simulink library "pack_5p48s8p_4g4g4_Thr_library"  (R2026a)
settings: Solver=VariableStepAuto
undefined symbols (not defined in the file or in its folder): batt_5p48s_1g10g1_thr, batt_5p48s_4g4g4_thr, battery_builder_rtmsupport, gcbh, ModuleAssembly1, ModuleType1, plate_5p48s_4g4g4_thr, targets_5p48s8p_4g4g4_thr
libraries: $bdroot x24, batt_lib x17, cooling_system_components x10, pack_5p48s8p_4g4g4_Thr_lib x4, fl_lib x1
Description:
  | Copyright 2023-2026 The MathWorks, Inc.
settings Model: Creator=smiller  LastModifiedBy=smiller

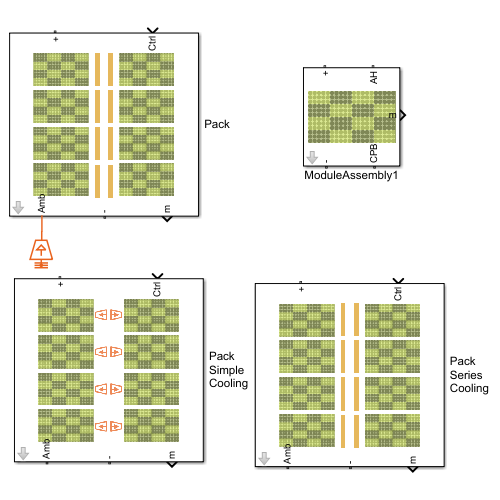
[thumbnail: Simulink's stored preview of the top-level diagram]
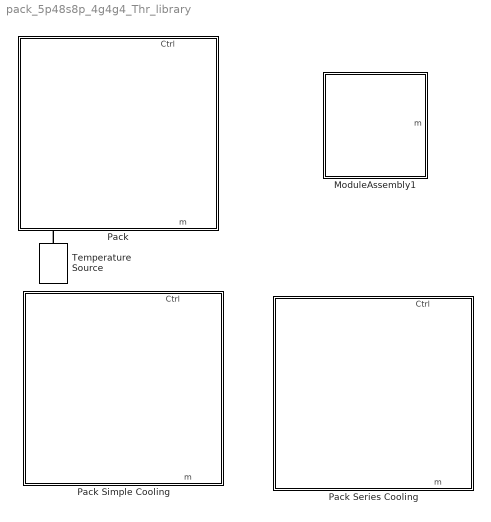
== system pack_5p48s8p_4g4g4_Thr_library ==
  ModuleAssembly1 : Subsystem  LoadFcn=battery_builder_rtmsupport('loadfcn',gcbh);  mask{Cell=ModuleType1, Targets=ModuleAssembly1, BatteryObj=batt_5p48s_1g10g1_thr}
      mask prompts: Cell "Cell Parameters"; Targets "Cell Targets"; BatteryObj "Battery Object"
      settings: PreCopyFcn=battery_builder_rtmsupport('precopyfcn',gcbh);  PreDeleteFcn=battery_builder_rtmsupport('predeletefcn',gcbh);  PortSchema="{\"entries\":[{\"content\":{\"sides\":[{\"content\":{\"connectorIds\":[\"LConn1\",\"LConn2\"]},\"type\":\"ConnectorPlacement.EquallySpacedRectSide\",\"uuid\":\"bc91a472-35c0-4041-89a6-b649b08794f0\"},{\"content\":{\"connectorIds\":[\"RConn1\",\"RConn2\"],\"side\":\"RIGHT\"},\"type\":\"ConnectorPlacement.EquallySpacedRectSide\",\"uuid\":\"4a390b53-12a2-4d2f-9537-abc76db307f8\"},{\"content\":{\"connectorIds\":[],\"side\":\"TOP\"},\"type\":\"ConnectorPlacement.EquallySpacedRectSide\",\"uuid\":\"1a7ed896-4ada-4d88-995c-c24bd39ee86b\"},{\"content\":{\"connectorIds\":[\"Out1\"],\"side\":\"BOTTOM\"},\"type\":\"ConnectorPlacement.EquallySpacedRectSide\",\"uuid\":\"e36c911b-adc9-44cf-bfab-32777b2ec35c\"}]},\"type\":\"ConnectorPlacement.EquallySpacedConnector\",\"uuid\":\"4e67d65b-f12d-4d00-91b0-7eadb0a42625\"}],\"packageUris\":[\"http://schema.mathworks.com/mf0/Connector/R2020b\"],\"version\":\"1.0\"}"
      mask Display: image('module_5p48s_4g4g4_IMAGE.png')
  Pack : Subsystem  LoadFcn=battery_builder_rtmsupport('loadfcn',gcbh);  mask{cell_param=ModuleType1, targets=targets_5p48s8p_4g4g4_thr, plate=plate_5p48s_4g4g4_thr, batt_obj=batt_5p48s_4g4g4_thr}
      mask prompts: cell_param "Cell Parameters"; targets "Cell Targets"; plate "Plate Parameters"; batt_obj "Battery Object"
      settings: PreCopyFcn=battery_builder_rtmsupport('precopyfcn',gcbh);  PreDeleteFcn=battery_builder_rtmsupport('predeletefcn',gcbh);
      mask Display: image('pack_5p48s8p_4g4g4_plate_IMAGE.png')
  Pack Series Cooling : Subsystem  LoadFcn=battery_builder_rtmsupport('loadfcn',gcbh);  mask{cell_param=ModuleType1, targets=targets_5p48s8p_4g4g4_thr, plate=plate_5p48s_4g4g4_thr, batt_obj=batt_5p48s_4g4g4_thr}
      mask prompts: cell_param "Cell Parameters"; targets "Cell Targets"; plate "Plate Parameters"; batt_obj "Battery Object"
      settings: PreCopyFcn=battery_builder_rtmsupport('precopyfcn',gcbh);  PreDeleteFcn=battery_builder_rtmsupport('predeletefcn',gcbh);
      mask Display: image('pack_5p48s8p_4g4g4_plate_IMAGE.png')
  Pack Simple Cooling : Subsystem  LoadFcn=battery_builder_rtmsupport('loadfcn',gcbh);  mask{cell_param=ModuleType1, targets=targets_5p48s8p_4g4g4_thr, plate=plate_5p48s_4g4g4_thr, batt_obj=batt_5p48s_4g4g4_thr, coolant_temp=[23 25]}
      mask prompts: cell_param "Cell Parameters"; targets "Cell Targets"; plate "Plate Parameters"; batt_obj "Battery Object"; coolant_temp "Coolant Temperature [In, Out] (degC)"
      settings: PreCopyFcn=battery_builder_rtmsupport('precopyfcn',gcbh);  PreDeleteFcn=battery_builder_rtmsupport('predeletefcn',gcbh);
      mask Display: image('pack_5p48s8p_4g4g4_bcnd_IMAGE.png')
  Temperature Source : fl_lib/Thermal/Thermal Sources/Temperature Source  temperature=298 K
  connections:
  Temperature Source/LConn1 -- Pack/RConn2

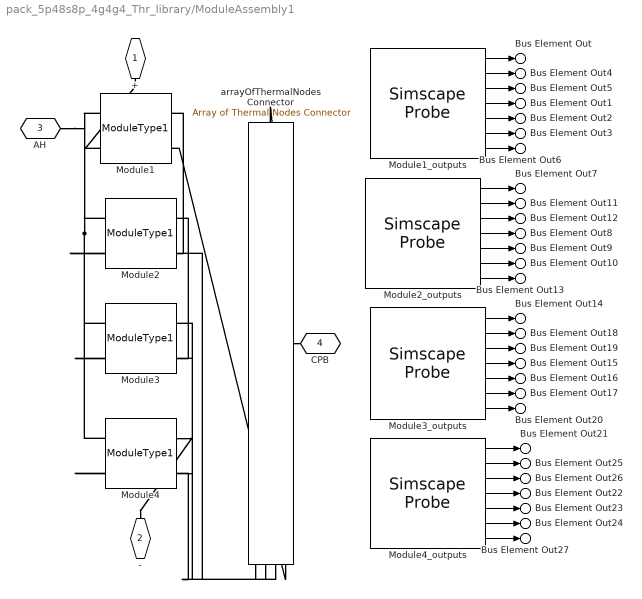
== system pack_5p48s8p_4g4g4_Thr_library/ModuleAssembly1 ==
  Module1 : pack_5p48s8p_4g4g4_Thr_lib/Modules/ModuleType1  BatteryCapacityCell=ModuleType1.BatteryCapacityCell A*hr  ExtrapolationMethodCell=simscape.enum.extrapolation.nearest  SOCBreakpointsCell=ModuleType1.SOCBreakpointsCell  TemperatureBreakpointsCell=ModuleType1.TemperatureBreakpointsCell K  OpenCircuitVoltageThermalCell=ModuleType1.OpenCircuitVoltageThermalCell V  VoltageRangeCell=ModuleType1.VoltageRangeCell V  ResistanceSOCBreakpointsCell=ModuleType1.ResistanceSOCBreakpointsCell  ResistanceTemperatureBreakpointsCell=ModuleType1.ResistanceTemperatureBreakpointsCell K  R0ThermalCell=ModuleType1.R0ThermalCell Ohm  BatteryThermalMassCell=ModuleType1.BatteryThermalMassCell J/K  CoolantResistance=Cell.CoolantResistance K/W  AmbientResistance=Cell.AmbientResistance K/W  socCell_specify=off  socCell_priority=High  socCell=repmat(1, 3, 1)  socCell_nominal_specify=off  socCell_nominal_value=1  socCell_nominal_unit=1  batteryVoltage_specify=off  batteryVoltage_priority=None  batteryVoltage=repmat(0, 3, 1) V  batteryVoltage_nominal_specify=off  batteryVoltage_nominal_value=1  batteryVoltage_nominal_unit=V  batteryCurrent_specify=off  batteryCurrent_priority=None  batteryCurrent=repmat(0, 3, 1) A  batteryCurrent_nominal_specify=off  batteryCurrent_nominal_value=1  batteryCurrent_nominal_unit=A  numCycles_specify=off  numCycles_priority=High  numCycles=repmat(0, 3, 1)  numCycles_nominal_specify=off  numCycles_nominal_value=1  numCycles_nominal_unit=1  batteryTemperature_specify=off  batteryTemperature_priority=High  batteryTemperature=repmat(298.15, 3, 1) K  batteryTemperature_nominal_specify=off  batteryTemperature_nominal_value=1  batteryTemperature_nominal_unit=K  vParallelAssembly_specify=on  vParallelAssembly_priority=None  vParallelAssembly=Targets.Module1.vParallelAssembly V  vParallelAssembly_nominal_specify=off  vParallelAssembly_nominal_value=1  vParallelAssembly_nominal_unit=V  socParallelAssembly_specify=on  socParallelAssembly_priority=None  socParallelAssembly=Targets.Module1.socParallelAssembly  socParallelAssembly_nominal_specify=off  socParallelAssembly_nominal_value=1  socParallelAssembly_nominal_unit=1
  Module1_outputs : SimscapeProbe  BoundBlock=1177  Variables="{\"batteryCurrent\":{\"Probing\":\"ON\"},\"batteryTemperature\":{\"Probing\":\"ON\"},\"batteryVoltage\":{\"Probing\":\"ON\"},\"iCell\":{\"Probing\":\"OFF\"},\"numCycles\":{\"Probing\":\"ON\"},\"numCyclesCell\":{\"Probing\":\"OFF\"},\"socCell\":{\"Probing\":\"ON\"},\"socParallelAssembly\":{\"Probing\":\"ON\"},\"temperatureCell\":{\"Probing\":\"OFF\"},\"vCell\":{\"Probing\":\"OFF\"},\"vParallelAssembly\":{\"Probing\":\"ON\"}}"
  Module2 : pack_5p48s8p_4g4g4_Thr_lib/Modules/ModuleType1  BatteryCapacityCell=ModuleType1.BatteryCapacityCell A*hr  ExtrapolationMethodCell=simscape.enum.extrapolation.nearest  SOCBreakpointsCell=ModuleType1.SOCBreakpointsCell  TemperatureBreakpointsCell=ModuleType1.TemperatureBreakpointsCell K  OpenCircuitVoltageThermalCell=ModuleType1.OpenCircuitVoltageThermalCell V  VoltageRangeCell=ModuleType1.VoltageRangeCell V  ResistanceSOCBreakpointsCell=ModuleType1.ResistanceSOCBreakpointsCell  ResistanceTemperatureBreakpointsCell=ModuleType1.ResistanceTemperatureBreakpointsCell K  R0ThermalCell=ModuleType1.R0ThermalCell Ohm  BatteryThermalMassCell=ModuleType1.BatteryThermalMassCell J/K  CoolantResistance=Cell.CoolantResistance K/W  AmbientResistance=Cell.AmbientResistance K/W  socCell_specify=off  socCell_priority=High  socCell=repmat(1, 3, 1)  socCell_nominal_specify=off  socCell_nominal_value=1  socCell_nominal_unit=1  batteryVoltage_specify=off  batteryVoltage_priority=None  batteryVoltage=repmat(0, 3, 1) V  batteryVoltage_nominal_specify=off  batteryVoltage_nominal_value=1  batteryVoltage_nominal_unit=V  batteryCurrent_specify=off  batteryCurrent_priority=None  batteryCurrent=repmat(0, 3, 1) A  batteryCurrent_nominal_specify=off  batteryCurrent_nominal_value=1  batteryCurrent_nominal_unit=A  numCycles_specify=off  numCycles_priority=High  numCycles=repmat(0, 3, 1)  numCycles_nominal_specify=off  numCycles_nominal_value=1  numCycles_nominal_unit=1  batteryTemperature_specify=off  batteryTemperature_priority=High  batteryTemperature=repmat(298.15, 3, 1) K  batteryTemperature_nominal_specify=off  batteryTemperature_nominal_value=1  batteryTemperature_nominal_unit=K  vParallelAssembly_specify=on  vParallelAssembly_priority=None  vParallelAssembly=Targets.Module2.vParallelAssembly V  vParallelAssembly_nominal_specify=off  vParallelAssembly_nominal_value=1  vParallelAssembly_nominal_unit=V  socParallelAssembly_specify=on  socParallelAssembly_priority=None  socParallelAssembly=Targets.Module2.socParallelAssembly  socParallelAssembly_nominal_specify=off  socParallelAssembly_nominal_value=1  socParallelAssembly_nominal_unit=1
  Module2_outputs : SimscapeProbe  BoundBlock=1178  Variables="{\"batteryCurrent\":{\"Probing\":\"ON\"},\"batteryTemperature\":{\"Probing\":\"ON\"},\"batteryVoltage\":{\"Probing\":\"ON\"},\"iCell\":{\"Probing\":\"OFF\"},\"numCycles\":{\"Probing\":\"ON\"},\"numCyclesCell\":{\"Probing\":\"OFF\"},\"socCell\":{\"Probing\":\"ON\"},\"socParallelAssembly\":{\"Probing\":\"ON\"},\"temperatureCell\":{\"Probing\":\"OFF\"},\"vCell\":{\"Probing\":\"OFF\"},\"vParallelAssembly\":{\"Probing\":\"ON\"}}"
  Module3 : pack_5p48s8p_4g4g4_Thr_lib/Modules/ModuleType1  BatteryCapacityCell=ModuleType1.BatteryCapacityCell A*hr  ExtrapolationMethodCell=simscape.enum.extrapolation.nearest  SOCBreakpointsCell=ModuleType1.SOCBreakpointsCell  TemperatureBreakpointsCell=ModuleType1.TemperatureBreakpointsCell K  OpenCircuitVoltageThermalCell=ModuleType1.OpenCircuitVoltageThermalCell V  VoltageRangeCell=ModuleType1.VoltageRangeCell V  ResistanceSOCBreakpointsCell=ModuleType1.ResistanceSOCBreakpointsCell  ResistanceTemperatureBreakpointsCell=ModuleType1.ResistanceTemperatureBreakpointsCell K  R0ThermalCell=ModuleType1.R0ThermalCell Ohm  BatteryThermalMassCell=ModuleType1.BatteryThermalMassCell J/K  CoolantResistance=Cell.CoolantResistance K/W  AmbientResistance=Cell.AmbientResistance K/W  socCell_specify=off  socCell_priority=High  socCell=repmat(1, 3, 1)  socCell_nominal_specify=off  socCell_nominal_value=1  socCell_nominal_unit=1  batteryVoltage_specify=off  batteryVoltage_priority=None  batteryVoltage=repmat(0, 3, 1) V  batteryVoltage_nominal_specify=off  batteryVoltage_nominal_value=1  batteryVoltage_nominal_unit=V  batteryCurrent_specify=off  batteryCurrent_priority=None  batteryCurrent=repmat(0, 3, 1) A  batteryCurrent_nominal_specify=off  batteryCurrent_nominal_value=1  batteryCurrent_nominal_unit=A  numCycles_specify=off  numCycles_priority=High  numCycles=repmat(0, 3, 1)  numCycles_nominal_specify=off  numCycles_nominal_value=1  numCycles_nominal_unit=1  batteryTemperature_specify=off  batteryTemperature_priority=High  batteryTemperature=repmat(298.15, 3, 1) K  batteryTemperature_nominal_specify=off  batteryTemperature_nominal_value=1  batteryTemperature_nominal_unit=K  vParallelAssembly_specify=on  vParallelAssembly_priority=None  vParallelAssembly=Targets.Module3.vParallelAssembly V  vParallelAssembly_nominal_specify=off  vParallelAssembly_nominal_value=1  vParallelAssembly_nominal_unit=V  socParallelAssembly_specify=on  socParallelAssembly_priority=None  socParallelAssembly=Targets.Module3.socParallelAssembly  socParallelAssembly_nominal_specify=off  socParallelAssembly_nominal_value=1  socParallelAssembly_nominal_unit=1
  Module3_outputs : SimscapeProbe  BoundBlock=1179  Variables="{\"batteryCurrent\":{\"Probing\":\"ON\"},\"batteryTemperature\":{\"Probing\":\"ON\"},\"batteryVoltage\":{\"Probing\":\"ON\"},\"iCell\":{\"Probing\":\"OFF\"},\"numCycles\":{\"Probing\":\"ON\"},\"numCyclesCell\":{\"Probing\":\"OFF\"},\"socCell\":{\"Probing\":\"ON\"},\"socParallelAssembly\":{\"Probing\":\"ON\"},\"temperatureCell\":{\"Probing\":\"OFF\"},\"vCell\":{\"Probing\":\"OFF\"},\"vParallelAssembly\":{\"Probing\":\"ON\"}}"
  Module4 : pack_5p48s8p_4g4g4_Thr_lib/Modules/ModuleType1  BatteryCapacityCell=ModuleType1.BatteryCapacityCell A*hr  ExtrapolationMethodCell=simscape.enum.extrapolation.nearest  SOCBreakpointsCell=ModuleType1.SOCBreakpointsCell  TemperatureBreakpointsCell=ModuleType1.TemperatureBreakpointsCell K  OpenCircuitVoltageThermalCell=ModuleType1.OpenCircuitVoltageThermalCell V  VoltageRangeCell=ModuleType1.VoltageRangeCell V  ResistanceSOCBreakpointsCell=ModuleType1.ResistanceSOCBreakpointsCell  ResistanceTemperatureBreakpointsCell=ModuleType1.ResistanceTemperatureBreakpointsCell K  R0ThermalCell=ModuleType1.R0ThermalCell Ohm  BatteryThermalMassCell=ModuleType1.BatteryThermalMassCell J/K  CoolantResistance=Cell.CoolantResistance K/W  AmbientResistance=Cell.AmbientResistance K/W  socCell_specify=off  socCell_priority=High  socCell=repmat(1, 3, 1)  socCell_nominal_specify=off  socCell_nominal_value=1  socCell_nominal_unit=1  batteryVoltage_specify=off  batteryVoltage_priority=None  batteryVoltage=repmat(0, 3, 1) V  batteryVoltage_nominal_specify=off  batteryVoltage_nominal_value=1  batteryVoltage_nominal_unit=V  batteryCurrent_specify=off  batteryCurrent_priority=None  batteryCurrent=repmat(0, 3, 1) A  batteryCurrent_nominal_specify=off  batteryCurrent_nominal_value=1  batteryCurrent_nominal_unit=A  numCycles_specify=off  numCycles_priority=High  numCycles=repmat(0, 3, 1)  numCycles_nominal_specify=off  numCycles_nominal_value=1  numCycles_nominal_unit=1  batteryTemperature_specify=off  batteryTemperature_priority=High  batteryTemperature=repmat(298.15, 3, 1) K  batteryTemperature_nominal_specify=off  batteryTemperature_nominal_value=1  batteryTemperature_nominal_unit=K  vParallelAssembly_specify=on  vParallelAssembly_priority=None  vParallelAssembly=Targets.Module4.vParallelAssembly V  vParallelAssembly_nominal_specify=off  vParallelAssembly_nominal_value=1  vParallelAssembly_nominal_unit=V  socParallelAssembly_specify=on  socParallelAssembly_priority=None  socParallelAssembly=Targets.Module4.socParallelAssembly  socParallelAssembly_nominal_specify=off  socParallelAssembly_nominal_value=1  socParallelAssembly_nominal_unit=1
  Module4_outputs : SimscapeProbe  BoundBlock=1180  Variables="{\"batteryCurrent\":{\"Probing\":\"ON\"},\"batteryTemperature\":{\"Probing\":\"ON\"},\"batteryVoltage\":{\"Probing\":\"ON\"},\"iCell\":{\"Probing\":\"OFF\"},\"numCycles\":{\"Probing\":\"ON\"},\"numCyclesCell\":{\"Probing\":\"OFF\"},\"socCell\":{\"Probing\":\"ON\"},\"socParallelAssembly\":{\"Probing\":\"ON\"},\"temperatureCell\":{\"Probing\":\"OFF\"},\"vCell\":{\"Probing\":\"OFF\"},\"vParallelAssembly\":{\"Probing\":\"ON\"}}"
  arrayOfThermalNodesConnector : batt_lib/Thermal/Array of Thermal Nodes Connector  numInputConnections=simscape.battery.enum.thermal.numArrayOfNodesConnections.four  concatenateDimension=2  complementaryDimensionsSize=1  inNode1NumElements=BatteryObj.Module(1).NumModels  inNode2NumElements=BatteryObj.Module(2).NumModels  inNode3NumElements=BatteryObj.Module(3).NumModels  inNode4NumElements=BatteryObj.Module(4).NumModels  inNode5NumElements=1  inNode6NumElements=1  inNode7NumElements=1  inNode8NumElements=1  inNode9NumElements=1  inNode10NumElements=1  inNode11NumElements=1  inNode12NumElements=1  inNode13NumElements=1  inNode14NumElements=1  inNode15NumElements=1  inNode16NumElements=1  inNode17NumElements=1  inNode18NumElements=1  inNode19NumElements=1  inNode20NumElements=1  inNode21NumElements=1  inNode22NumElements=1  inNode23NumElements=1  inNode24NumElements=1  inNode25NumElements=1  inNode26NumElements=1  inNode27NumElements=1  inNode28NumElements=1  inNode29NumElements=1  inNode30NumElements=1  inNode31NumElements=1  inNode32NumElements=1  inNode33NumElements=1  inNode34NumElements=1  inNode35NumElements=1  inNode36NumElements=1  inNode37NumElements=1  inNode38NumElements=1  inNode39NumElements=1  inNode40NumElements=1  inNode41NumElements=1  inNode42NumElements=1  inNode43NumElements=1  inNode44NumElements=1  inNode45NumElements=1  inNode46NumElements=1  inNode47NumElements=1  inNode48NumElements=1  inNode49NumElements=1  inNode50NumElements=1
  + : PMIOPort  Side=Left
  - : PMIOPort  Port=2  Side=Right
  AH : PMIOPort  Port=3  Side=Left
  CPB : PMIOPort  Port=4  Side=Right
  Bus Element Out : Outport  PortName=m  Element=i.M1
  Bus Element Out7 : Outport  PortName=m  Element=i.M2
  Bus Element Out14 : Outport  PortName=m  Element=i.M3
  Bus Element Out21 : Outport  PortName=m  Element=i.M4
  Bus Element Out1 : Outport  PortName=m  Element=cyc.M1
  Bus Element Out8 : Outport  PortName=m  Element=cyc.M2
  Bus Element Out15 : Outport  PortName=m  Element=cyc.M3
  Bus Element Out22 : Outport  PortName=m  Element=cyc.M4
  Bus Element Out2 : Outport  PortName=m  Element=socC.M1
  Bus Element Out9 : Outport  PortName=m  Element=socC.M2
  Bus Element Out16 : Outport  PortName=m  Element=socC.M3
  Bus Element Out23 : Outport  PortName=m  Element=socC.M4
  Bus Element Out3 : Outport  PortName=m  Element=socP.M1
  Bus Element Out10 : Outport  PortName=m  Element=socP.M2
  Bus Element Out17 : Outport  PortName=m  Element=socP.M3
  Bus Element Out24 : Outport  PortName=m  Element=socP.M4
  Bus Element Out4 : Outport  PortName=m  Element=T.M1
  Bus Element Out11 : Outport  PortName=m  Element=T.M2
  Bus Element Out18 : Outport  PortName=m  Element=T.M3
  Bus Element Out25 : Outport  PortName=m  Element=T.M4
  Bus Element Out5 : Outport  PortName=m  Element=vC.M1
  Bus Element Out12 : Outport  PortName=m  Element=vC.M2
  Bus Element Out19 : Outport  PortName=m  Element=vC.M3
  Bus Element Out26 : Outport  PortName=m  Element=vC.M4
  Bus Element Out6 : Outport  PortName=m  Element=vP.M1
  Bus Element Out13 : Outport  PortName=m  Element=vP.M2
  Bus Element Out20 : Outport  PortName=m  Element=vP.M3
  Bus Element Out27 : Outport  PortName=m  Element=vP.M4
  wires:
  Module1_outputs/1 -> Bus Element Out/1
  Module1_outputs/2 -> Bus Element Out4/1
  Module1_outputs/3 -> Bus Element Out5/1
  Module1_outputs/4 -> Bus Element Out1/1
  Module1_outputs/5 -> Bus Element Out2/1
  Module1_outputs/6 -> Bus Element Out3/1
  Module1_outputs/7 -> Bus Element Out6/1
  Module2_outputs/1 -> Bus Element Out7/1
  Module2_outputs/2 -> Bus Element Out11/1
  Module2_outputs/3 -> Bus Element Out12/1
  Module2_outputs/4 -> Bus Element Out8/1
  Module2_outputs/5 -> Bus Element Out9/1
  Module2_outputs/6 -> Bus Element Out10/1
  Module2_outputs/7 -> Bus Element Out13/1
  Module3_outputs/1 -> Bus Element Out14/1
  Module3_outputs/2 -> Bus Element Out18/1
  Module3_outputs/3 -> Bus Element Out19/1
  Module3_outputs/4 -> Bus Element Out15/1
  Module3_outputs/5 -> Bus Element Out16/1
  Module3_outputs/6 -> Bus Element Out17/1
  Module3_outputs/7 -> Bus Element Out20/1
  Module4_outputs/1 -> Bus Element Out21/1
  Module4_outputs/2 -> Bus Element Out25/1
  Module4_outputs/3 -> Bus Element Out26/1
  Module4_outputs/4 -> Bus Element Out22/1
  Module4_outputs/5 -> Bus Element Out23/1
  Module4_outputs/6 -> Bus Element Out24/1
  Module4_outputs/7 -> Bus Element Out27/1
  connections:
  Module2/LConn2 -- Module1/RConn1
  Module3/LConn2 -- Module2/RConn1
  Module4/LConn2 -- Module3/RConn1
  Module1/LConn2 -- +/RConn1
  Module4/RConn1 -- -/RConn1
  Module4/LConn1 -- Module3/LConn1 -- Module2/LConn1 -- Module1/LConn1 -- AH/RConn1
  arrayOfThermalNodesConnector/LConn2 -- Module3/RConn2
  arrayOfThermalNodesConnector/LConn4 -- Module1/RConn2
  arrayOfThermalNodesConnector/LConn3 -- Module2/RConn2
  arrayOfThermalNodesConnector/RConn1 -- CPB/RConn1
  arrayOfThermalNodesConnector/LConn1 -- Module4/RConn2

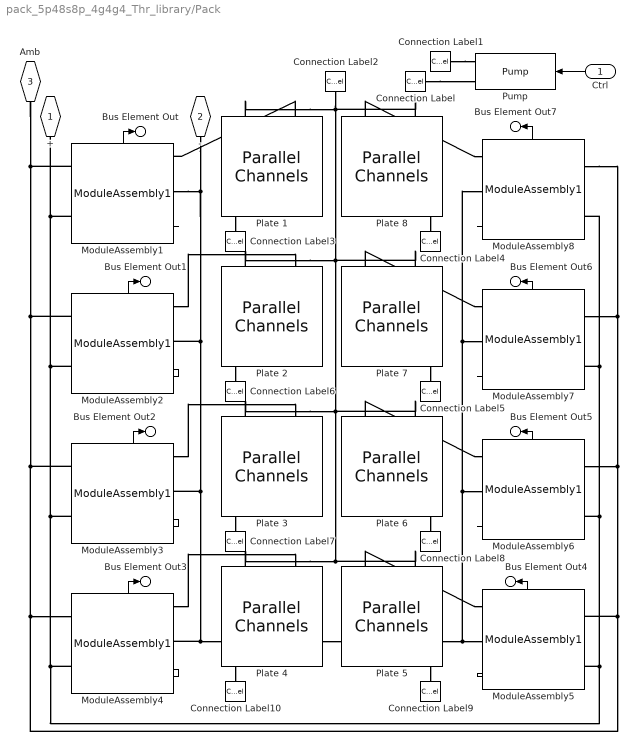
== system pack_5p48s8p_4g4g4_Thr_library/Pack ==
  Ctrl : Inport
  Connection Label : ConnectionLabel  Label=Plate
  Connection Label{1,3..10} (9 alike) : ConnectionLabel  Label=Return
  Connection Label2 : ConnectionLabel  Label=Plate
  ModuleAssembly1 : $bdroot/ModuleAssembly1  Cell=cell_param  Targets=targets.ModuleAssembly1  BatteryObj=batt_obj
  ModuleAssembly2 : $bdroot/ModuleAssembly1  Cell=cell_param  Targets=targets.ModuleAssembly2  BatteryObj=batt_obj
  ModuleAssembly3 : $bdroot/ModuleAssembly1  Cell=cell_param  Targets=targets.ModuleAssembly3  BatteryObj=batt_obj
  ModuleAssembly4 : $bdroot/ModuleAssembly1  Cell=cell_param  Targets=targets.ModuleAssembly4  BatteryObj=batt_obj
  ModuleAssembly5 : $bdroot/ModuleAssembly1  Cell=cell_param  Targets=targets.ModuleAssembly5  BatteryObj=batt_obj
  ModuleAssembly6 : $bdroot/ModuleAssembly1  Cell=cell_param  Targets=targets.ModuleAssembly6  BatteryObj=batt_obj
  ModuleAssembly7 : $bdroot/ModuleAssembly1  Cell=cell_param  Targets=targets.ModuleAssembly7  BatteryObj=batt_obj
  ModuleAssembly8 : $bdroot/ModuleAssembly1  Cell=cell_param  Targets=targets.ModuleAssembly8  BatteryObj=batt_obj
  Plate {1..8} (8 alike) : batt_lib/Thermal/Parallel Channels  plateConnectivity=simscape.battery.enum.thermal.coolingPlateConnectivity.singleSided  numBattThermalNodes1=plate.Nodes  dimensionThermalNodes1=plate.Dimensions  locationThermalNodes1=plate.Coordinates  numBattThermalNodes2=1  dimensionThermalNodes2=ones(1, 2)  locationThermalNodes2=ones(1, 2)  plateDimX=plate.partitions_x  plateDimY=plate.partitions_y  plateTh=plate.thickness m  plateThCond=plate.k_thermal W/(K*m)  plateDen=plate.rho kg/m^3  plateCp=plate.cp J/(K*kg)  plateTemp_ini=plate.coolant_temp K  Re_lam=2000  Re_tur=4000  Nu_lam=3.66  length_add=1e-3 m  shape_factor=64  nChannels=plate.num_channels  selectChannelOrientation=simscape.battery.enum.thermal.coolingChannelsDirection.alongX  channelDia=plate.diameter_hyd m  distributorDia=plate.diameter_dst m  roughnessPipe=plate.pipe_rough m
  Pump : cooling_system_components/Pump  num_plates=8
  + : PMIOPort  Side=Left
  - : PMIOPort  Port=2  Side=Right
  Amb : PMIOPort  Port=3  Side=Right
  Bus Element Out : Outport  PortName=m  Element=A1
  Bus Element Out1 : Outport  PortName=m  Element=A2
  Bus Element Out2 : Outport  PortName=m  Element=A3
  Bus Element Out3 : Outport  PortName=m  Element=A4
  Bus Element Out4 : Outport  PortName=m  Element=A5
  Bus Element Out5 : Outport  PortName=m  Element=A6
  Bus Element Out6 : Outport  PortName=m  Element=A7
  Bus Element Out7 : Outport  PortName=m  Element=A8
  wires:
  ModuleAssembly1/1 -> Bus Element Out/1
  ModuleAssembly2/1 -> Bus Element Out1/1
  ModuleAssembly3/1 -> Bus Element Out2/1
  ModuleAssembly4/1 -> Bus Element Out3/1
  ModuleAssembly5/1 -> Bus Element Out4/1
  ModuleAssembly6/1 -> Bus Element Out5/1
  ModuleAssembly7/1 -> Bus Element Out6/1
  ModuleAssembly8/1 -> Bus Element Out7/1
  Ctrl/1 -> Pump/1
  connections:
  Amb/RConn1 -- ModuleAssembly1/LConn2 -- ModuleAssembly2/LConn2 -- ModuleAssembly7/LConn2 -- ModuleAssembly8/LConn2 -- ModuleAssembly6/LConn2 -- ModuleAssembly5/LConn2 -- ModuleAssembly4/LConn2 -- ModuleAssembly3/LConn2
  ModuleAssembly1/RConn1 -- -/RConn1 -- ModuleAssembly2/RConn1 -- ModuleAssembly3/RConn1 -- ModuleAssembly4/RConn1 -- ModuleAssembly8/RConn1 -- ModuleAssembly7/RConn1 -- ModuleAssembly6/RConn1 -- ModuleAssembly5/RConn1
  ModuleAssembly1/LConn1 -- ModuleAssembly4/LConn1 -- ModuleAssembly6/LConn1 -- ModuleAssembly8/LConn1 -- ModuleAssembly7/LConn1 -- ModuleAssembly5/LConn1 -- ModuleAssembly3/LConn1 -- ModuleAssembly2/LConn1 -- +/RConn1
  ModuleAssembly3/RConn2 -- Plate 3/LConn2
  ModuleAssembly2/RConn2 -- Plate 2/LConn2
  ModuleAssembly4/RConn2 -- Plate 4/LConn2
  Plate 1/LConn2 -- ModuleAssembly1/RConn2
  Plate 7/LConn2 -- ModuleAssembly7/RConn2
  Plate 6/LConn2 -- ModuleAssembly6/RConn2
  Plate 5/LConn2 -- ModuleAssembly5/RConn2
  Plate 8/LConn2 -- ModuleAssembly8/RConn2
  Connection Label2/LConn1 -- Plate 1/LConn1 -- Plate 8/LConn1 -- Plate 7/LConn1 -- Plate 2/LConn1 -- Plate 3/LConn1 -- Plate 6/LConn1 -- Plate 5/LConn1 -- Plate 4/LConn1
  Plate 2/RConn1 -- Connection Label6/LConn1
  Plate 3/RConn1 -- Connection Label7/LConn1
  Connection Label1/LConn1 -- Pump/RConn1
  Plate 4/RConn1 -- Connection Label10/LConn1
  Plate 8/RConn1 -- Connection Label4/LConn1
  Plate 6/RConn1 -- Connection Label8/LConn1
  Plate 1/RConn1 -- Connection Label3/LConn1
  Plate 7/RConn1 -- Connection Label5/LConn1
  Plate 5/RConn1 -- Connection Label9/LConn1
  Connection Label/LConn1 -- Pump/RConn2

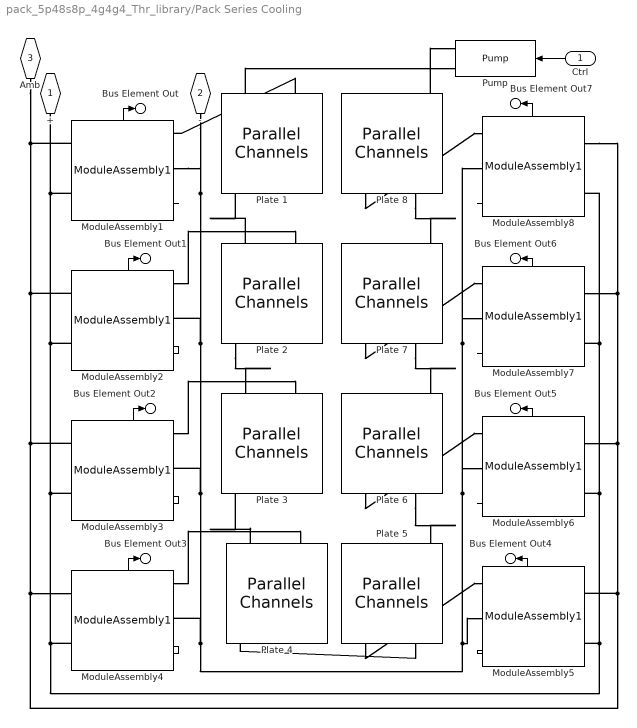
== system pack_5p48s8p_4g4g4_Thr_library/Pack Series Cooling ==
  Ctrl : Inport
  ModuleAssembly1 : $bdroot/ModuleAssembly1  Cell=cell_param  Targets=targets.ModuleAssembly1  BatteryObj=batt_obj
  ModuleAssembly2 : $bdroot/ModuleAssembly1  Cell=cell_param  Targets=targets.ModuleAssembly2  BatteryObj=batt_obj
  ModuleAssembly3 : $bdroot/ModuleAssembly1  Cell=cell_param  Targets=targets.ModuleAssembly3  BatteryObj=batt_obj
  ModuleAssembly4 : $bdroot/ModuleAssembly1  Cell=cell_param  Targets=targets.ModuleAssembly4  BatteryObj=batt_obj
  ModuleAssembly5 : $bdroot/ModuleAssembly1  Cell=cell_param  Targets=targets.ModuleAssembly5  BatteryObj=batt_obj
  ModuleAssembly6 : $bdroot/ModuleAssembly1  Cell=cell_param  Targets=targets.ModuleAssembly6  BatteryObj=batt_obj
  ModuleAssembly7 : $bdroot/ModuleAssembly1  Cell=cell_param  Targets=targets.ModuleAssembly7  BatteryObj=batt_obj
  ModuleAssembly8 : $bdroot/ModuleAssembly1  Cell=cell_param  Targets=targets.ModuleAssembly8  BatteryObj=batt_obj
  Plate {1..8} (8 alike) : batt_lib/Thermal/Parallel Channels  plateConnectivity=simscape.battery.enum.thermal.coolingPlateConnectivity.singleSided  numBattThermalNodes1=plate.Nodes  dimensionThermalNodes1=plate.Dimensions  locationThermalNodes1=plate.Coordinates  numBattThermalNodes2=1  dimensionThermalNodes2=ones(1, 2)  locationThermalNodes2=ones(1, 2)  plateDimX=plate.partitions_x  plateDimY=plate.partitions_y  plateTh=plate.thickness m  plateThCond=plate.k_thermal W/(K*m)  plateDen=plate.rho kg/m^3  plateCp=plate.cp J/(K*kg)  plateTemp_ini=plate.coolant_temp K  Re_lam=2000  Re_tur=4000  Nu_lam=3.66  length_add=1e-3 m  shape_factor=64  nChannels=plate.num_channels  selectChannelOrientation=simscape.battery.enum.thermal.coolingChannelsDirection.alongX  channelDia=plate.diameter_hyd m  distributorDia=plate.diameter_dst m  roughnessPipe=plate.pipe_rough m
  Pump : cooling_system_components/Pump  num_plates=8
  + : PMIOPort  Side=Left
  - : PMIOPort  Port=2  Side=Right
  Amb : PMIOPort  Port=3  Side=Right
  Bus Element Out : Outport  PortName=m  Element=A1
  Bus Element Out1 : Outport  PortName=m  Element=A2
  Bus Element Out2 : Outport  PortName=m  Element=A3
  Bus Element Out3 : Outport  PortName=m  Element=A4
  Bus Element Out4 : Outport  PortName=m  Element=A5
  Bus Element Out5 : Outport  PortName=m  Element=A6
  Bus Element Out6 : Outport  PortName=m  Element=A7
  Bus Element Out7 : Outport  PortName=m  Element=A8
  wires:
  Ctrl/1 -> Pump/1
  ModuleAssembly8/1 -> Bus Element Out7/1
  ModuleAssembly7/1 -> Bus Element Out6/1
  ModuleAssembly6/1 -> Bus Element Out5/1
  ModuleAssembly5/1 -> Bus Element Out4/1
  ModuleAssembly4/1 -> Bus Element Out3/1
  ModuleAssembly3/1 -> Bus Element Out2/1
  ModuleAssembly2/1 -> Bus Element Out1/1
  ModuleAssembly1/1 -> Bus Element Out/1
  connections:
  Plate 8/RConn1 -- Pump/RConn1
  Plate 1/LConn1 -- Pump/RConn2
  Plate 8/LConn2 -- ModuleAssembly8/RConn2
  Plate 5/LConn2 -- ModuleAssembly5/RConn2
  Plate 6/LConn2 -- ModuleAssembly6/RConn2
  Plate 7/LConn2 -- ModuleAssembly7/RConn2
  Plate 1/LConn2 -- ModuleAssembly1/RConn2
  Plate 2/RConn1 -- Plate 3/LConn1
  ModuleAssembly4/RConn2 -- Plate 4/LConn2
  Plate 5/LConn1 -- Plate 4/RConn1
  Plate 8/LConn1 -- Plate 7/RConn1
  ModuleAssembly2/RConn2 -- Plate 2/LConn2
  Plate 2/LConn1 -- Plate 1/RConn1
  Plate 7/LConn1 -- Plate 6/RConn1
  Plate 6/LConn1 -- Plate 5/RConn1
  ModuleAssembly3/RConn2 -- Plate 3/LConn2
  Plate 4/LConn1 -- Plate 3/RConn1
  +/RConn1 -- ModuleAssembly2/LConn1 -- ModuleAssembly3/LConn1 -- ModuleAssembly5/LConn1 -- ModuleAssembly7/LConn1 -- ModuleAssembly8/LConn1 -- ModuleAssembly6/LConn1 -- ModuleAssembly4/LConn1 -- ModuleAssembly1/LConn1
  ModuleAssembly5/RConn1 -- ModuleAssembly6/RConn1 -- ModuleAssembly7/RConn1 -- ModuleAssembly8/RConn1 -- ModuleAssembly4/RConn1 -- ModuleAssembly3/RConn1 -- ModuleAssembly2/RConn1 -- -/RConn1 -- ModuleAssembly1/RConn1
  ModuleAssembly3/LConn2 -- ModuleAssembly4/LConn2 -- ModuleAssembly5/LConn2 -- ModuleAssembly6/LConn2 -- ModuleAssembly8/LConn2 -- ModuleAssembly7/LConn2 -- ModuleAssembly2/LConn2 -- ModuleAssembly1/LConn2 -- Amb/RConn1

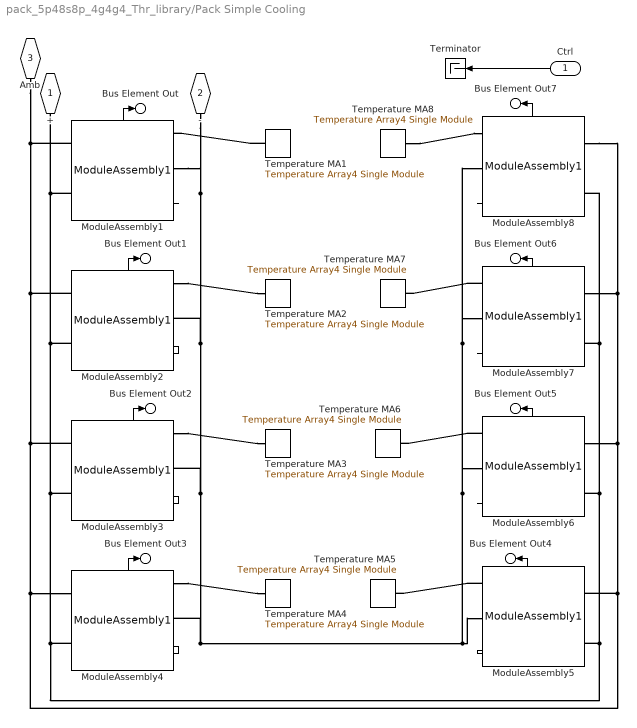
== system pack_5p48s8p_4g4g4_Thr_library/Pack Simple Cooling ==
  Ctrl : Inport
  ModuleAssembly1 : $bdroot/ModuleAssembly1  Cell=cell_param  Targets=targets.ModuleAssembly1  BatteryObj=batt_obj
  ModuleAssembly2 : $bdroot/ModuleAssembly1  Cell=cell_param  Targets=targets.ModuleAssembly2  BatteryObj=batt_obj
  ModuleAssembly3 : $bdroot/ModuleAssembly1  Cell=cell_param  Targets=targets.ModuleAssembly3  BatteryObj=batt_obj
  ModuleAssembly4 : $bdroot/ModuleAssembly1  Cell=cell_param  Targets=targets.ModuleAssembly4  BatteryObj=batt_obj
  ModuleAssembly5 : $bdroot/ModuleAssembly1  Cell=cell_param  Targets=targets.ModuleAssembly5  BatteryObj=batt_obj
  ModuleAssembly6 : $bdroot/ModuleAssembly1  Cell=cell_param  Targets=targets.ModuleAssembly6  BatteryObj=batt_obj
  ModuleAssembly7 : $bdroot/ModuleAssembly1  Cell=cell_param  Targets=targets.ModuleAssembly7  BatteryObj=batt_obj
  ModuleAssembly8 : $bdroot/ModuleAssembly1  Cell=cell_param  Targets=targets.ModuleAssembly8  BatteryObj=batt_obj
  Temperature MA{1..8} (8 alike) : cooling_system_components/Temperature Array4 Single Module  t_in=coolant_temp(1)  t_out=coolant_temp(2)
  Terminator : Terminator
  + : PMIOPort  Side=Left
  - : PMIOPort  Port=2  Side=Right
  Amb : PMIOPort  Port=3  Side=Right
  Bus Element Out : Outport  PortName=m  Element=A1
  Bus Element Out1 : Outport  PortName=m  Element=A2
  Bus Element Out2 : Outport  PortName=m  Element=A3
  Bus Element Out3 : Outport  PortName=m  Element=A4
  Bus Element Out4 : Outport  PortName=m  Element=A5
  Bus Element Out5 : Outport  PortName=m  Element=A6
  Bus Element Out6 : Outport  PortName=m  Element=A7
  Bus Element Out7 : Outport  PortName=m  Element=A8
  wires:
  ModuleAssembly8/1 -> Bus Element Out7/1
  ModuleAssembly7/1 -> Bus Element Out6/1
  ModuleAssembly6/1 -> Bus Element Out5/1
  ModuleAssembly5/1 -> Bus Element Out4/1
  ModuleAssembly4/1 -> Bus Element Out3/1
  ModuleAssembly3/1 -> Bus Element Out2/1
  ModuleAssembly2/1 -> Bus Element Out1/1
  ModuleAssembly1/1 -> Bus Element Out/1
  Ctrl/1 -> Terminator/1
  connections:
  Temperature MA8/LConn1 -- ModuleAssembly8/RConn2
  Temperature MA1/LConn1 -- ModuleAssembly1/RConn2
  +/RConn1 -- ModuleAssembly2/LConn1 -- ModuleAssembly3/LConn1 -- ModuleAssembly5/LConn1 -- ModuleAssembly7/LConn1 -- ModuleAssembly8/LConn1 -- ModuleAssembly6/LConn1 -- ModuleAssembly4/LConn1 -- ModuleAssembly1/LConn1
  ModuleAssembly5/RConn1 -- ModuleAssembly6/RConn1 -- ModuleAssembly7/RConn1 -- ModuleAssembly8/RConn1 -- ModuleAssembly4/RConn1 -- ModuleAssembly3/RConn1 -- ModuleAssembly2/RConn1 -- -/RConn1 -- ModuleAssembly1/RConn1
  ModuleAssembly3/LConn2 -- ModuleAssembly4/LConn2 -- ModuleAssembly5/LConn2 -- ModuleAssembly6/LConn2 -- ModuleAssembly8/LConn2 -- ModuleAssembly7/LConn2 -- ModuleAssembly2/LConn2 -- ModuleAssembly1/LConn2 -- Amb/RConn1
  ModuleAssembly5/RConn2 -- Temperature MA5/LConn1
  ModuleAssembly6/RConn2 -- Temperature MA6/LConn1
  ModuleAssembly3/RConn2 -- Temperature MA3/LConn1
  ModuleAssembly7/RConn2 -- Temperature MA7/LConn1
  ModuleAssembly2/RConn2 -- Temperature MA2/LConn1
  ModuleAssembly4/RConn2 -- Temperature MA4/LConn1
